simulink model "StreetLaneSegment2x2"  (R2021a)
settings: Solver=VariableStepAuto  StartTime=0.0  StopTime=10.0  RelTol=1e-3
undefined symbols (not defined in the file): Kz, Tz
settings Model: Creator=phill  LastModifiedBy=phill

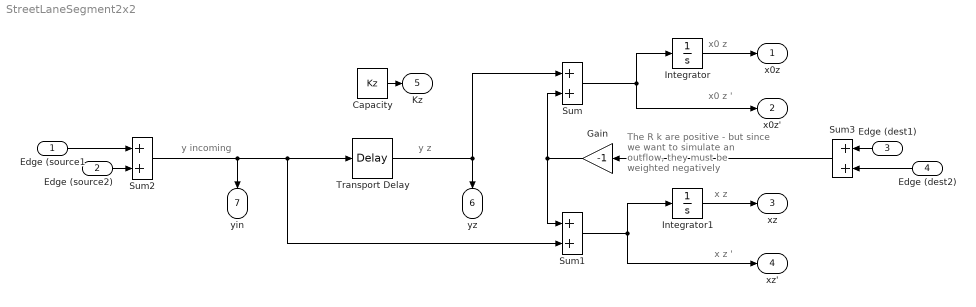
== system StreetLaneSegment2x2 ==
  note: x0 z
  note: The R k are positive - but since we
      | want to simulate an outflow, they
      | must be weighted negatively
  note: y incoming
  note: x z
  note: x0 z '
  note: x z '
  note: y z
  Edge (source1 : Inport
  Edge (source2) : Inport  Port=2
  Edge (dest1) : Inport  Port=3
  Edge (dest2) : Inport  Port=4
  Capacity : Constant  Value=Kz
  Gain : Gain  Gain=-1
  Integrator : Integrator
  Integrator1 : Integrator
  Sum{,1..3} (4 alike) : Sum
  Transport Delay : TransportDelay  DelayTime=Tz
  x0z : Outport
  x0z' : Outport  Port=2
  xz : Outport  Port=3
  xz' : Outport  Port=4
  Kz : Outport  Port=5
  yz : Outport  Port=6
  yin : Outport  Port=7
  wires:
  Gain/1 -> Sum1/1, Sum/2
  Sum1/1 -> xz'/1, Integrator1/1
  Sum/1 -> Integrator/1, x0z'/1
  Transport Delay/1 -> yz/1, Sum/1
  Sum2/1 -> yin/1, Sum1/2, Transport Delay/1
  Sum3/1 -> Gain/1
  Integrator1/1 -> xz/1
  Integrator/1 -> x0z/1
  Capacity/1 -> Kz/1
  Edge (source1/1 -> Sum2/1
  Edge (source2)/1 -> Sum2/2
  Edge (dest1)/1 -> Sum3/1
  Edge (dest2)/1 -> Sum3/2
